simulink model "dingdiankongzhi"  (R2016a)
settings: Solver=VariableStepAuto  StartTime=0.0  StopTime=10.0  RelTol=1e-3
undefined symbols (not defined in the file): Angular, Linear
libraries: simulink x4, robotlib x3
settings Model: Creator=Wangkuo  LastModifiedBy=Wangkuo
settings GRTTargetCC: GeneratePreprocessorConditionals=Use local settings

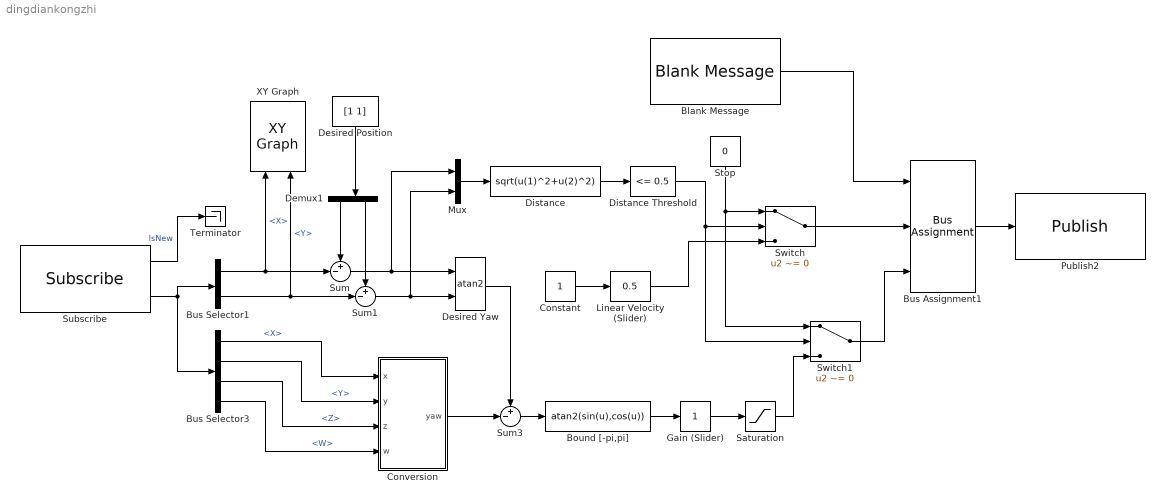
== system dingdiankongzhi ==
  Blank Message : robotlib/Blank Message  SourceLibraryInfo=This block requires Robotics System Toolbox  messageType=geometry_msgs/Twist  SampleTime=inf
  Bound [-pi,pi] : Fcn  Expr=atan2(sin(u),cos(u))
  Bus Assignment1 : BusAssignment  DialogController=Simulink.DDGSource_BusAssignment  AssignedSignals=Linear.X,Angular.Z
  Bus Selector1 : BusSelector  OutputSignals=Pose.Pose.Position.X,Pose.Pose.Position.Y
  Bus Selector3 : BusSelector  OutputSignals=Pose.Pose.Orientation.X,Pose.Pose.Orientation.Y,Pose.Pose.Orientation.Z,Pose.Pose.Orientation.W
  Constant : Constant
  Conversion : MATLAB Function  TreatAsAtomicUnit=on
  Demux1 : Demux  Outputs=2
  Desired Position : Constant  Value=[1 1]
  Desired Yaw : Trigonometry  Operator=atan2
  Distance : Fcn  Expr=sqrt(u(1)^2+u(2)^2)
  Distance Threshold : simulink/Logic and Bit Operations/Compare To Constant  relop=<=  const=0.5  OutDataTypeStr=boolean
  Gain (Slider) : simulink/Math Operations/Slider Gain  low=1  gain=1  high=3
  Linear Velocity (Slider) : simulink/Math Operations/Slider Gain  low=0  gain=0.5  high=1
  Mux : Mux  Inputs=2
  Publish2 : robotlib/Publish  SourceLibraryInfo=This block requires Robotics System Toolbox  topicSource=Select from ROS network  topic=/mobile_base/commands/velocity  messageType=geometry_msgs/Twist  messageQueueLength=105
  Saturation : Saturate
  Stop : Constant  Value=0
  Subscribe : robotlib/Subscribe  SourceLibraryInfo=This block requires Robotics System Toolbox  topicSource=Select from ROS network  topic=/odom  messageType=nav_msgs/Odometry  sampleTime=-1  messageQueueLength=51
  Sum : Sum  Inputs=+-|
  Sum1 : Sum  Inputs=+-|
  Sum3 : Sum  Inputs=+-|
  Switch : Switch  Criteria=u2 ~= 0
  Switch1 : Switch  Criteria=u2 ~= 0
  Terminator : Terminator
  XY Graph : simulink/Sinks/XY Graph  xmin=-1  xmax=1  ymin=-1  ymax=1  st=-1
  wires:
  Subscribe/2 -> Bus Selector3/1, Bus Selector1/1
  Bus Selector3/1 -> Conversion/1(x)  "<X>"
  Bus Selector3/2 -> Conversion/2(y)  "<Y>"
  Bus Selector3/3 -> Conversion/3(z)  "<Z>"
  Bus Selector3/4 -> Conversion/4(w)  "<W>"
  Bus Selector1/2 -> Sum1/2, XY Graph/2  "<Y>"
  Bus Selector1/1 -> Sum/2, XY Graph/1  "<X>"
  Linear Velocity (Slider)/1 -> Switch/3
  Sum3/1 -> Bound [-pi,pi]/1
  Stop/1 -> Switch1/1, Switch/1
  Saturation/1 -> Switch1/3
  Gain (Slider)/1 -> Saturation/1
  Distance Threshold/1 -> Switch/2, Switch1/2
  Sum/1 -> Desired Yaw/1, Mux/1
  Desired Yaw/1 -> Sum3/1
  Conversion/1(yaw) -> Sum3/2
  Bound [-pi,pi]/1 -> Gain (Slider)/1
  Mux/1 -> Distance/1
  Distance/1 -> Distance Threshold/1
  Desired Position/1 -> Demux1/1
  Constant/1 -> Linear Velocity (Slider)/1
  Sum1/1 -> Desired Yaw/2, Mux/2
  Demux1/2 -> Sum1/1
  Demux1/1 -> Sum/1
  Switch1/1 -> Bus Assignment1/3
  Switch/1 -> Bus Assignment1/2
  Blank Message/1 -> Bus Assignment1/1
  Bus Assignment1/1 -> Publish2/1
  Subscribe/1 -> Terminator/1  "IsNew"

== matlab function dingdiankongzhi/Conversion ==
  data: yaw output; x input; y input; z input; w input
function yaw  = quat2eul(x,y,z,w)
%#codegen

% Convert the quaternion to a yaw angle (zyx euler angle)
eul = quat2eul([w,x,y,z]);
yaw = eul(1);

end
